simulink model "Sim_model"  (Simulink 8.4)
settings: Solver=ode45  StartTime=0.0  StopTime=110  RelTol=1e-3
libraries: fuzblock x2, simulink x1
CloseFcn:
  | rtwprivate ssgensfun ModelCloseRequest nlgentpl
settings Model: Creator=lbusoniu  LastModifiedBy=Nikhil  ExtModeAutoUpdateStatusClock=off  BufferReuse=off
settings DataIOCC: SaveOutput=off  SaveTime=off  SignalLoggingName=sigsOut
settings OptimizationCC: OptimizeBlockIOStorage=off  BufferReuse=off  GlobalBufferReuse=off  ExpressionFolding=off  ExpressionDepthLimit=128  LocalBlockOutputs=off  InitFltsAndDblsToZero=on
settings DebuggingCC: SaveWithParameterizedLinksMsg=none  SignalResolutionControl=TryResolveAllWithWarning  SolverPrmCheckMsg=none  MultiTaskDSMMsg=warning  MultiTaskCondExecSysMsg=none  StateNameClashWarn=none
settings HardwareCC: TargetUnknown=on
settings RTWCC: IncludeERTFirstTime=on
settings GRTTargetCC: TargetFcnLib=ansi_tfl_tmw.mat

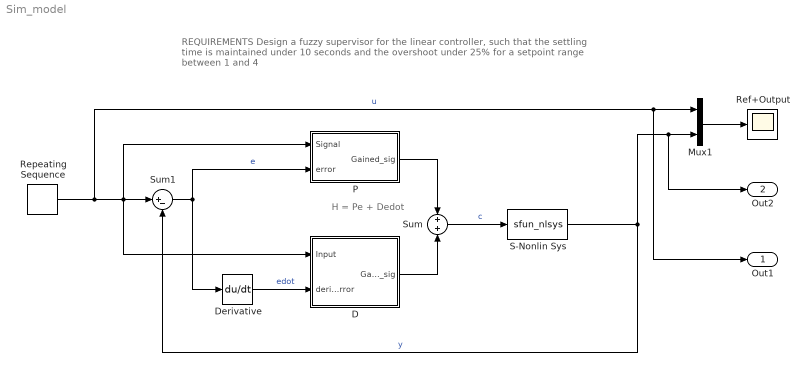
== system Sim_model ==
  note: H = Pe + Dedot
  note: REQUIREMENTS
      | Design a fuzzy supervisor for the linear controller, such that
      | the settling time is maintained under 10 seconds and the overshoot under 25%
      | for a setpoint range between 1 and 4
  D : Subsystem
  Derivative : Derivative
  Mux1 : Mux  Inputs=2
  P : Subsystem
  Ref+Output : Scope
      settings: TimeRange=110  YMin=0.5  YMax=1.1  SaveName=out
  Repeating Sequence : simulink/Sources/Repeating Sequence  rep_seq_t=[0 15 15.5 30 30.5 45 45.5 60 60.5 75 75.5 90 91.5 111]  rep_seq_y=[1 1 .5 .5 2 2 1.5 1.5 3 3 2.5 2.5 4 4]
  S-Nonlin Sys : S-Function  FunctionName=sfun_nlsys  EnableBusSupport=off
  Sum : Sum
  Sum1 : Sum  Inputs=|+-  SaturateOnIntegerOverflow=on
  Out1 : Outport
  Out2 : Outport  Port=2
  wires:
  S-Nonlin Sys/1 -> Out2/1, Mux1/2, Sum1/2  "y"
  Mux1/1 -> Ref+Output/1
  Repeating Sequence/1 -> Sum1/1, P/1(Signal), D/1(Input), Out1/1, Mux1/1  "u"
  P/1(Gained_sig) -> Sum/1
  Sum1/1 -> Derivative/1, P/2(error)  "e"
  Derivative/1 -> D/2(derivative error)  "edot"
  D/1(Gained_sig) -> Sum/2
  Sum/1 -> S-Nonlin Sys/1  "c"

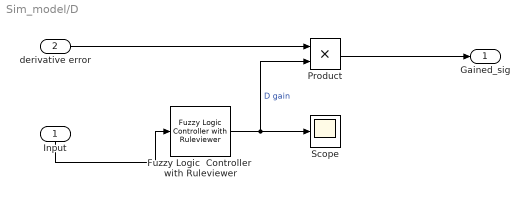
== system Sim_model/D ==
  Input : Inport
  derivative error : Inport  Port=2
  Fuzzy Logic  Controller  with Ruleviewer : fuzblock/Fuzzy Logic  Controller  with Ruleviewer  fismatrix=derivative  Ts=110
  Product : Product
  Scope : Scope
  Gained_sig : Outport
  wires:
  Input/1 -> Fuzzy Logic  Controller  with Ruleviewer/1
  derivative error/1 -> Product/1
  Fuzzy Logic  Controller  with Ruleviewer/1 -> Product/2, Scope/1  "D gain"
  Product/1 -> Gained_sig/1

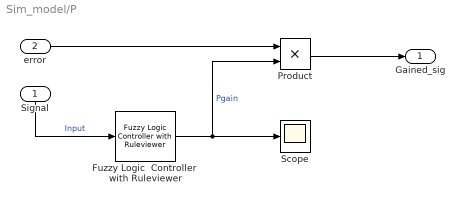
== system Sim_model/P ==
  Signal : Inport
  error : Inport  Port=2
  Fuzzy Logic  Controller  with Ruleviewer : fuzblock/Fuzzy Logic  Controller  with Ruleviewer  fismatrix=proportional  Ts=110
  Product : Product
  Scope : Scope
  Gained_sig : Outport
  wires:
  Signal/1 -> Fuzzy Logic  Controller  with Ruleviewer/1  "Input"
  error/1 -> Product/1
  Fuzzy Logic  Controller  with Ruleviewer/1 -> Product/2, Scope/1  "Pgain"
  Product/1 -> Gained_sig/1
